simulink model "Prescan_Carsim_0118_repair_cs"  (R2019b)
settings: Solver=ode5  StartTime=0.0  StopTime=inf  FixedStep=1/1000  RelTol=1e-3
PreLoadFcn:
  | mbxruntime.callbacks.PreLoadFcn(bdroot);
PostLoadFcn:
  | mbxruntime.callbacks.PostLoadFcn(bdroot);
InitFcn:
  | mbxruntime.callbacks.InitFcn(bdroot);
  | Initialization_Func;
  | %T01_Init_2106;
StartFcn:
  | mbxruntime.callbacks.StartFcn(bdroot);
  | current_sys=gcs;
  | speedblock=Simulink.findBlocks(current_sys,'Name','speed_kmh_Gain');
  | h1=add_exec_event_listener(speedblock,'PostOutputs',@SpeedVisulization);
  | outblock=Simulink.findBlocks(current_sys,'Name','trajectorycurveoutput_Gain');
  | CurveTrajectoryListenerHandle=add_exec_event_listener(outblock,'PostOutputs',@TrajectoryCurve_CallBack);
  | lanedatablock=Simulink.findBlocks(current_sys,'Name','LaneData_Gain');
  | CurveLaneListenerHandle=add_exec_event_listener(lanedatablock,'PostOutputs',@CurveLane_CallBack);
StopFcn:
  | mbxruntime.callbacks.StopFcn(bdroot);
model workspace: external: MAT-File .\Prescan_Carsim_1230_cs_hws.mat (data not in the file)
undefined symbols (not defined in the file or in its folder): AAx, AAy, AAz, AVx, AVy, AVz, Ax, Ay, Az, canChannel, DiscIntNeverNeededParam, g, InitialDPMPDF_Comfort, InitialDPMPDF_Efficiency, InitialDPMPDF_Safety, InitialPDF_DEM, InitialPlanningParameter, Kf, Kr, Lr, M, mbxruntime, nG, NormalisedTrajectoryIndicator_Pool, Parameter_Indicator_LookUpTable, Prescan_Carsim_1230_cs_0658e9ca1334a8be, Prescan_Carsim_1230_cs_08c5eb9a1bd7376a, Prescan_Carsim_1230_cs_6cfd759b89b9fc85, Prescan_Carsim_1230_cs_9435cc1cceb5050d, Prescan_Carsim_1230_cs_ac716d34d49f74ab, Prescan_Carsim_1230_cs_be02757d7f212dd5, Rational_Coefficient_Learning, SteeringWheel, TrajectoryIndicatorRange, V, VehicleBaseLength, Vx, Vy, Vz, WheelL0, WheelL1, WheelR0, WheelR1
libraries: canmsglib x11, dsparch4 x6, canlib x3, PreScanSimulinkLibrary x3, Solver_SF x1, autolibshared x1
(part 2 of 8)

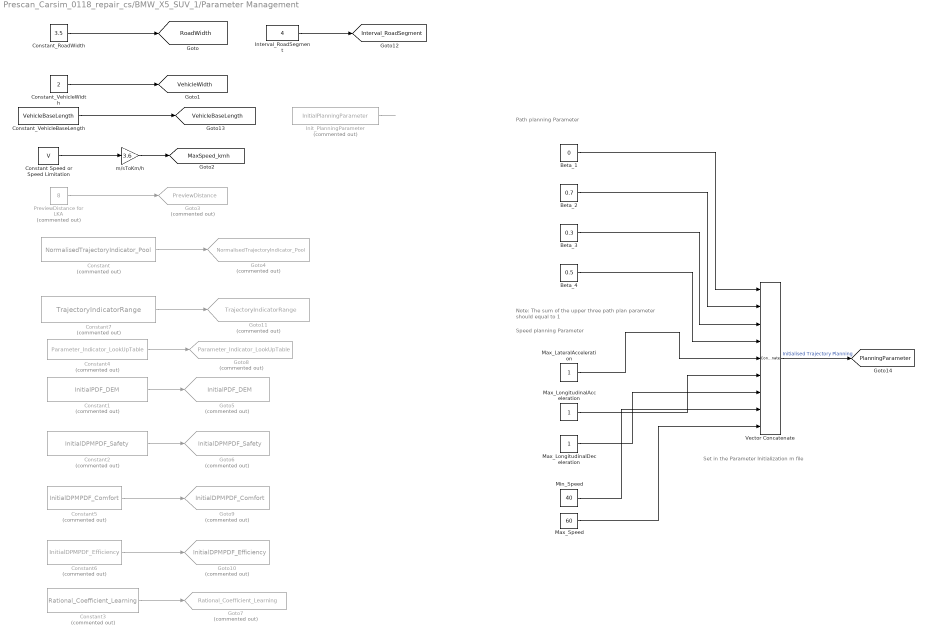
== system Prescan_Carsim_0118_repair_cs/BMW_X5_SUV_1/Parameter Management ==
  note: Set in the Parameter Initialization m file
  note: Note: The sum of the upper three path plan parameter should equal to 1
  note: Speed planning Parameter
  note: Path planning Parameter
  Beta_1 : Constant  Value=0
      settings: AttributesFormatString=|
      | weight of short path
      | within 0-1
  Beta_2 : Constant  Value=0.7
      settings: AttributesFormatString=|
      | weight of minimum curvature path
      | within 0-1
  Beta_3 : Constant  Value=0.3
      settings: AttributesFormatString=|
      | weight of fixed lateral offset
      | within 0-1
  Beta_4 : Constant  Value=0.5
      settings: AttributesFormatString=Fixed lateral offset distance
  Constant : Constant  Commented=on  Value=NormalisedTrajectoryIndicator_Pool
  Constant Speed or Speed Limitation : Constant  Value=V
  Constant1 : Constant  Commented=on  Value=InitialPDF_DEM
      settings: AttributesFormatString=|
      | The Initial probability density Distribution
      | of the S-C-E weight of the DEM
  Constant2 : Constant  Commented=on  Value=InitialDPMPDF_Safety
      settings: AttributesFormatString=|
      | The Initial probability density Distribution
      | of the DPM for S-C-E
  Constant3 : Constant  Commented=on  Value=Rational_Coefficient_Learning
  Constant4 : Constant  Commented=on  Value=Parameter_Indicator_LookUpTable
  Constant5 : Constant  Commented=on  Value=InitialDPMPDF_Comfort
      settings: AttributesFormatString=|
      | The Initial probability density Distribution
      | of the DPM for S-C-E
  Constant6 : Constant  Commented=on  Value=InitialDPMPDF_Efficiency
      settings: AttributesFormatString=|
      | The Initial probability density Distribution
      | of the DPM for S-C-E
  Constant7 : Constant  Commented=on  Value=TrajectoryIndicatorRange
  Constant_RoadWidth : Constant  Value=3.5
  Constant_VehicleBaseLength : Constant  Value=VehicleBaseLength
  Constant_VehicleWidth : Constant  Value=2
  Goto10 : Goto  Commented=on  GotoTag=InitialDPMPDF_Efficiency  TagVisibility=global
  Goto11 : Goto  Commented=on  GotoTag=TrajectoryIndicatorRange  TagVisibility=global
  Goto3 : Goto  Commented=on  GotoTag=PreviewDistance  TagVisibility=global
  Goto4 : Goto  Commented=on  GotoTag=NormalisedTrajectoryIndicator_Pool  TagVisibility=global
  Goto5 : Goto  Commented=on  GotoTag=InitialPDF_DEM  TagVisibility=global
  Goto6 : Goto  Commented=on  GotoTag=InitialDPMPDF_Safety  TagVisibility=global
  Goto7 : Goto  Commented=on  GotoTag=Rational_Coefficient_Learning  TagVisibility=global
  Goto8 : Goto  Commented=on  GotoTag=Parameter_Indicator_LookUpTable  TagVisibility=global
  Goto9 : Goto  Commented=on  GotoTag=InitialDPMPDF_Comfort  TagVisibility=global
  Init_PlanningParameter : Constant  Commented=on  Value=InitialPlanningParameter
  Interval_RoadSegment : Constant  Value=4
  Max_LateralAcceleration : Constant
      settings: AttributesFormatString=|
      | Maximum Lateral Acceleration (m/s2)
      | (within 0.5-2.5)
  Max_LongitudinalAcceleration : Constant
      settings: AttributesFormatString=|
      | Maximum Longitudinal Acceleration(m/s2)
      | ((within 0-3))
  Max_LongitudinalDeceleration : Constant
      settings: AttributesFormatString=|
      | Maximum Longitudinal Deceleration(m/s2)
      | (within 0-3)
  Max_Speed : Constant  Value=60
      settings: AttributesFormatString=Alowable Maximum Speed (Km/h)
  Min_Speed : Constant  Value=40
      settings: AttributesFormatString=Alowable Minimum Speed (Km/h)
  PreviewDistance for LKA : Constant  Commented=on  Value=8
  Vector Concatenate : Concatenate  NumInputs=9  Mode=Multidimensional array
  m/sToKm/h : Gain  Gain=3.6
  tag scope: Interval_RoadSegment=global, MaxSpeed_kmh=global, PlanningParameter=global, RoadWidth=global, VehicleBaseLength=global, VehicleWidth=global
  wires:
  m/sToKm/h/1 -> [MaxSpeed_kmh]
  PreviewDistance for LKA/1 -> Goto3/1
  Constant Speed or Speed Limitation/1 -> m/sToKm/h/1
  Constant_VehicleWidth/1 -> [VehicleWidth]
  Constant_RoadWidth/1 -> [RoadWidth]
  Constant/1 -> Goto4/1
  Constant1/1 -> Goto5/1
  Constant2/1 -> Goto6/1
  Constant3/1 -> Goto7/1
  Constant4/1 -> Goto8/1
  Constant5/1 -> Goto9/1
  Constant6/1 -> Goto10/1
  Constant7/1 -> Goto11/1
  Max_Speed/1 -> Vector Concatenate/9
  Max_LateralAcceleration/1 -> Vector Concatenate/5
  Beta_2/1 -> Vector Concatenate/2
  Max_LongitudinalDeceleration/1 -> Vector Concatenate/7
  Max_LongitudinalAcceleration/1 -> Vector Concatenate/6
  Beta_4/1 -> Vector Concatenate/4
  Min_Speed/1 -> Vector Concatenate/8
  Beta_1/1 -> Vector Concatenate/1
  Beta_3/1 -> Vector Concatenate/3
  Vector Concatenate/1 -> [PlanningParameter]  "Initialised Trajectory Planning"
  Interval_RoadSegment/1 -> [Interval_RoadSegment]
  Constant_VehicleBaseLength/1 -> [VehicleBaseLength]
  Init_PlanningParameter/1 -> ?

== system Prescan_Carsim_0118_repair_cs/BMW_X5_SUV_1/SELF_Demux ==
  SELF : Inport  OutDataTypeStr=Bus: PRESCAN_SELFSENSORDATA
  Bus Selector : BusSelector  OutputSignals=PositionX,PositionY,PositionZ,OrientationRoll,OrientationPitch,OrientationYaw,Velocity,Yaw_rate,Lat,Long,Alt,TimeStamp
  Demux2 : Demux  Outputs=3
  Gain : Gain  Gain=180/pi
  Gain1 : Gain  Gain=180/pi
  Vector Concatenate1 : Concatenate  NumInputs=3
  compas converter : Subsystem
  x [m] : Outport
  y [m] : Outport  Port=2
  z [m] : Outport  Port=3
  rotx [deg] : Outport  Port=4
  roty [deg] : Outport  Port=5
  rotz [deg] : Outport  Port=6
  GPS lat [deg] : Outport  Port=7
  GPS long [deg] : Outport  Port=8
  GPS alt [m] : Outport  Port=9
  velocity [m/s] : Outport  Port=10
  heading [deg] : Outport  Port=11
  yaw rate [deg/s] : Outport  Port=12
  TimeStamp [s] : Outport  Port=13
  wires:
  Bus Selector/12 -> TimeStamp [s]/1  "<TimeStamp>"
  Bus Selector/11 -> GPS alt [m]/1  "<Alt>"
  Bus Selector/10 -> GPS long [deg]/1  "<Long>"
  Bus Selector/9 -> GPS lat [deg]/1  "<Lat>"
  Bus Selector/8 -> Gain1/1  "<Yaw_rate>"
  Bus Selector/7 -> velocity [m/s]/1  "<Velocity>"
  Bus Selector/6 -> compas converter/1(rotz [rad]), Vector Concatenate1/3  "<OrientationYaw>"
  Bus Selector/5 -> Vector Concatenate1/2  "<OrientationPitch>"
  Bus Selector/4 -> Vector Concatenate1/1  "<OrientationRoll>"
  Vector Concatenate1/1 -> Gain/1
  Bus Selector/3 -> z [m]/1  "<PositionZ>"
  Bus Selector/2 -> y [m]/1  "<PositionY>"
  Bus Selector/1 -> x [m]/1  "<PositionX>"
  SELF/1 -> Bus Selector/1
  Gain/1 -> Demux2/1
  Demux2/1 -> rotx [deg]/1
  Demux2/2 -> roty [deg]/1
  Demux2/3 -> rotz [deg]/1
  compas converter/1(heading [deg]) -> heading [deg]/1
  Gain1/1 -> yaw rate [deg/s]/1

== system Prescan_Carsim_0118_repair_cs/BMW_X5_SUV_1/STATE_BMW_X5_SUV_1 ==
  State : Inport  SampleTime=TimeStep
  Bus Creator : BusCreator  Inputs=15  OutDataTypeStr=Bus: PRESCAN_STATEACTUATORDATA  NonVirtualBus=on
  Constant : Constant  Value=0
  Demux : Demux  Outputs=15
  Mux : Mux  Inputs=3
  Mux1 : Mux  Inputs=3
  Mux2 : Mux  Inputs=3
  iniBODYAngles wrtVEH [rad] : Constant  Value=Roll0  SampleTime=TimeStep
  iniBODYAngles wrtVEH [rad]1 : Constant  Value=Pitch0  SampleTime=TimeStep
  iniVEHAngles wrtGLOB [rad] : Constant  Value=Yaw0  SampleTime=TimeStep
  iniVEHposition wrtGLOB [m] : Constant  Value=x0  SampleTime=TimeStep
  iniVEHposition wrtGLOB [m]1 : Constant  Value=y0  SampleTime=TimeStep
  iniVEHposition wrtGLOB [m]2 : Constant  Value=z0  SampleTime=TimeStep
  state2FullState : PreScanSimulinkLibrary/state2FullState  SystemSampleTime=-1  Latency=0  AutoFrameSizeCalculation=off
  StateBus : Outport  OutDataTypeStr=Bus: PRESCAN_STATEACTUATORDATA
  wires:
  Bus Creator/1 -> StateBus/1
  State/1 -> state2FullState/1
  state2FullState/1 -> Demux/1
  Demux/1 -> Bus Creator/1  "PositionX"
  Demux/2 -> Bus Creator/2  "PositionY"
  Demux/3 -> Bus Creator/3  "PositionZ"
  Demux/4 -> Bus Creator/4  "VelocityX"
  Demux/5 -> Bus Creator/5  "VelocityY"
  Demux/6 -> Bus Creator/6  "VelocityZ"
  Demux/7 -> Bus Creator/7  "AccelerationX"
  Demux/8 -> Bus Creator/8  "AccelerationY"
  Demux/9 -> Bus Creator/9  "AccelerationZ"
  Demux/10 -> Bus Creator/10  "OrientationRoll"
  Demux/11 -> Bus Creator/11  "OrientationPitch"
  Demux/12 -> Bus Creator/12  "OrientationYaw"
  Demux/13 -> Bus Creator/13  "AngularVelocityRoll"
  Demux/14 -> Bus Creator/14  "AngularVelocityPitch"
  Demux/15 -> Bus Creator/15  "AngularVelocityYaw"
  iniVEHposition wrtGLOB [m]1/1 -> Mux/2
  iniVEHposition wrtGLOB [m]/1 -> Mux/1
  iniVEHposition wrtGLOB [m]2/1 -> Mux/3
  Mux/1 -> state2FullState/2
  iniBODYAngles wrtVEH [rad]/1 -> Mux1/1
  iniBODYAngles wrtVEH [rad]1/1 -> Mux1/2
  Constant/1 -> Mux1/3, Mux2/2, Mux2/1
  Mux1/1 -> state2FullState/3
  iniVEHAngles wrtGLOB [rad]/1 -> Mux2/3
  Mux2/1 -> state2FullState/4

== system Prescan_Carsim_0118_repair_cs/BMW_X5_SUV_1/SteeringWheel_pivot_Mux ==
  X [m] : Inport
  Y [m] : Inport  Port=2
  Z [m] : Inport  Port=3
  Roll [rad] : Inport  Port=4
  Pitch [rad] : Inport  Port=5
  Yaw [rad] : Inport  Port=6
  Bus Creator : BusCreator  Inputs=3  OutDataTypeStr=Bus: PRESCAN_XYZ_DATA
  Bus Creator1 : BusCreator  Inputs=3  OutDataTypeStr=Bus: PRESCAN_RPY_DATA
  Bus Creator2 : BusCreator  Inputs=2  OutDataTypeStr=Bus: PRESCAN_POSE_DATA
  Joint : Outport
  wires:
  Yaw [rad]/1 -> Bus Creator1/3  "Yaw"
  Bus Creator1/1 -> Bus Creator2/2  "ORIENTATION"
  Bus Creator/1 -> Bus Creator2/1  "POSITION"
  X [m]/1 -> Bus Creator/1  "X"
  Y [m]/1 -> Bus Creator/2  "Y"
  Z [m]/1 -> Bus Creator/3  "Z"
  Bus Creator2/1 -> Joint/1
  Roll [rad]/1 -> Bus Creator1/1  "Roll"
  Pitch [rad]/1 -> Bus Creator1/2  "Pitch"

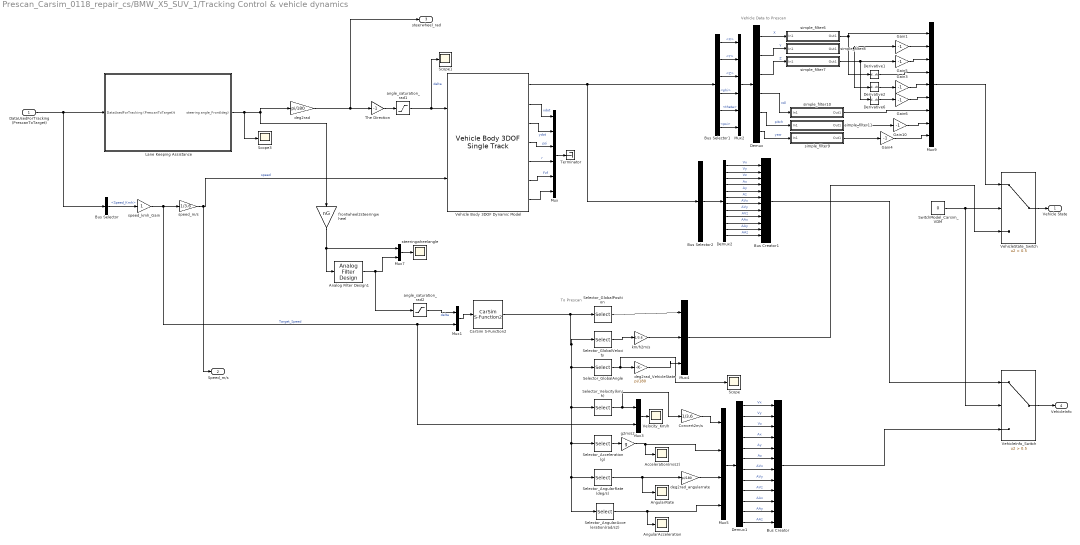
== system Prescan_Carsim_0118_repair_cs/BMW_X5_SUV_1/Tracking Control & vehicle dynamics ==
  note: To Prescan
  note: Vehicle Data to Prescan
  DataUsedForTracking (PrescanToTarget) : Inport
  Acceleration(m/s2) : Scope
  Analog Filter Design1 : dsparch4/Analog Filter Design  method=Butterworth  filttype=Lowpass  N=1  Wlo=5  Whi=80  Rp=2  Rs=40
  AngularAcceleration : Scope
  AngularRate : Scope
  Bus Creator : BusCreator  Inputs=Vx,Vy,Vz,Ax,Ay,Az,AVx,AVy,AVz,AAx,AAy,AAz
  Bus Creator1 : BusCreator  Inputs=Vx,Vy,Vz,Ax,Ay,Az,AVx,AVy,AVz,AAx,AAy,AAz
  Bus Selector : BusSelector  OutputSignals=Speed_Kmh
  Bus Selector1 : BusSelector  OutputSignals=InertFrm.Cg.Disp.X,InertFrm.Cg.Disp.Y,InertFrm.Cg.Disp.Z,InertFrm.Cg.Ang.phi,InertFrm.Cg.Ang.theta,InertFrm.Cg.Ang.psi
  Bus Selector2 : BusSelector  OutputSignals=BdyFrm.Cg.Vel.xdot,BdyFrm.Cg.Vel.ydot,BdyFrm.Cg.Vel.zdot,BdyFrm.Cg.Acc.xddot,BdyFrm.Cg.Acc.yddot,BdyFrm.Cg.Acc.zddot,BdyFrm.Cg.AngVel.p,BdyFrm.Cg.AngVel.q,BdyFrm.Cg.AngVel.r,BdyFrm.Cg.AngAcc.pdot,BdyFrm.Cg.AngAcc.qdot,BdyFrm.Cg.AngAcc.rdot  OutputAsBus=on
  CarSim S-Function2 : Solver_SF/CarSim S-Function2  Priority=1  VehicleCode=i_i  SIMFILE=simfile.sim
      settings: SourceProductName=CarSim S-Function
      settings: AttributesFormatString=|
      | Vehicle Code: %<VehicleCode>
      | Input:Steering Wheel Angel(deg)
      | 2,Speed(km/h)
      | Output:
      | 1,X,Y,Z(m)
      | 2,Roll,Pitch,Yaw(deg)
      | 3,Longitudinal and Lateral Acceleration(g)
      | 4,Roll,Pitch and Yaw rate (deg/s)
      | 5,Roll and Yaw acceleration (rad/s2)
      | 6,SteeringWheelAngel and 4 Wheels Angle(deg)
  Convert2m/s : Gain  Gain=1/3.6
  Demux : Demux  Outputs=6
  Demux1 : Demux  Outputs=12
  Demux2 : Demux  Outputs=12  BusSelectionMode=on
  Derivative1 : Derivative
  Derivative2 : Derivative
  Derivative6 : Derivative
  Gain{1,3..6,10} (6 alike) : Gain  Gain=-1
  Lane Keeping Assistance : Subsystem
  Mux : Mux  Inputs=6
  Mux1 : Mux  Inputs=2
  Mux2 : Mux  Inputs=6
  Mux3 : Mux  Inputs=2
  Mux4 : Mux  Inputs=3
  Mux5 : Mux
  Mux7 : Mux  Inputs=2
  Mux9 : Mux  Inputs=9
  Scope : Scope
  Scope1 : Scope
  Scope3 : Scope
  Selector_Acceleration(g) : Selector  InputPortWidth=21  IndexOptions=Index vector (dialog)  Indices=[13:15]  OutputSizes=1
  Selector_AngularAcceleration(rad/s2) : Selector  InputPortWidth=21  IndexOptions=Index vector (dialog)  Indices=[19:21]  OutputSizes=1
  Selector_AngularRate(deg/s) : Selector  InputPortWidth=21  IndexOptions=Index vector (dialog)  Indices=[16:18]  OutputSizes=1
  Selector_GlobalAngle : Selector  InputPortWidth=21  IndexOptions=Index vector (dialog)  Indices=[7:9]  OutputSizes=1
  Selector_GlobalPosition : Selector  InputPortWidth=21  IndexOptions=Index vector (dialog)  Indices=[1:3]  OutputSizes=1
  Selector_GlobalVelocity : Selector  InputPortWidth=21  IndexOptions=Index vector (dialog)  Indices=[4:6]  OutputSizes=1
  Selector_Velocity(km/h) : Selector  InputPortWidth=21  IndexOptions=Index vector (dialog)  Indices=[10:12]  OutputSizes=1
  SwitchModel_Carsim_VDM : Constant  Value=0
      settings: AttributesFormatString=|
      | 0:Carsim
      | 1:Simulink VDM
  Terminator : Terminator
  "The Direction " : Gain  Gain=-1
  Vehicle Body 3DOF Dynamic Model : autolibshared/Vehicle Body 3DOF Single Track  trackMode=Single (bicycle)  inputMode=External longitudinal velocity  frontSteerMode=on  rearSteerMode=off  windMode=off  muMode=off  extFMode=off  extMMode=off  extXo=off  extpsio=off  extxdoto=off  extro=off  extYo=off  extTamb=off  extydoto=off  aMode=2  NF=2  NR=2  m=M  a=Lf  b=Lr  h=0.35  X_o=0  xdot_o=0  CalphaMode=off  sigmaMode=off  d=0  w=[1.4,1.4]  Cy_f=Kf*2  Cy_r=Kr*2  sigma_f=.1  sigma_r=.1  alpha_f_brk=[-.1 .1]  Cy_f_data=[-9e3 9e3]  alpha_r_brk=[-.1 .1]  Cy_r_data=[-9e3 9e3]  Y_o=0  ydot_o=0  Izz=I  psi_o=0  r_o=0  Af=0  Cd=.3  Cl=.1  Cpm=.1  beta_w=[0:0.01:0.3]  Cs=[0:0.03:0.9]  Cym=[0:0.01:0.3]  Pabs=101325  Tair=273  g=g  mu=1  xdot_tol=.01  Fznom=5000  Fxtire_sat=7e4  Fytire_sat=7e4  longOff=0  latOff=0  vertOff=0  wrapAng=off
      settings: SourceProductBaseCode=PW,MT,VE,VP
  VehicleInfo_Switch : Switch  Criteria=u2 > Threshold  Threshold=0.5
  VehicleState_Switch : Switch  Criteria=u2 > Threshold  Threshold=0.5
  Velocity_Km/h : Scope
  angle_saturation_rad1 : Saturate  UpperLimit=1.5  LowerLimit=-1.5
  angle_saturation_rad2 : Saturate  UpperLimit=86  LowerLimit=-86
  deg2rad : Gain  Gain=pi/180
  deg2rad_VehicleState : Gain  Gain=pi/180
  deg2rad_angularrate : Gain  Gain=pi/180
  frontwheel2steeringwheel : Gain  Gain=nG
      settings: AttributesFormatString=Calculatedd by the carsim table
  g2m/s2 : Gain  Gain=g
  km/h2m/s : Gain  Gain=1/3.6
  simple_filter10 : Subsystem
  simple_filter11 : Subsystem
  simple_filter6 : Subsystem
  simple_filter7 : Subsystem
  simple_filter8 : Subsystem
  simple_filter9 : Subsystem
  speed_kmh_Gain : Gain
  speed_m/s : Gain  Gain=1/3.6
  steeringwheelangle : Scope
  Vehicle State : Outport
  Speed_m/s : Outport  Port=2
  "steerwheel_rad " : Outport  Port=3
  VehicleInfo : Outport  Port=4
  wires:
  "The Direction "/1 -> angle_saturation_rad1/1
  Mux/1 -> Terminator/1
  Vehicle Body 3DOF Dynamic Model/7 -> Mux/6
  Vehicle Body 3DOF Dynamic Model/6 -> Mux/5  "Fzf"
  Vehicle Body 3DOF Dynamic Model/5 -> Mux/4  "r"
  Vehicle Body 3DOF Dynamic Model/4 -> Mux/3  "psi"
  Vehicle Body 3DOF Dynamic Model/3 -> Mux/2  "ydot"
  Vehicle Body 3DOF Dynamic Model/2 -> Mux/1  "xdot"
  angle_saturation_rad1/1 -> Scope1/1, Vehicle Body 3DOF Dynamic Model/1  "delta"
  deg2rad/1 -> "steerwheel_rad "/1, "The Direction "/1
  DataUsedForTracking (PrescanToTarget)/1 -> Bus Selector/1, Lane Keeping Assistance/1(DataUsedForTracking (PrescanToTarget)t)
  Bus Selector1/3 -> Mux2/3  "<Z>"
  simple_filter9/1(Out1) -> Gain4/1
  Bus Selector1/5 -> Mux2/5  "<theta>"
  Gain4/1 -> Mux9/9
  Demux/5 -> simple_filter11/1(In1)  "pitch"
  simple_filter8/1(Out1) -> Derivative2/1, Gain1/1
  Demux/6 -> simple_filter9/1(In1)  "yaw"
  Gain6/1 -> Mux9/6
  simple_filter6/1(Out1) -> Derivative1/1, Mux9/1
  Gain1/1 -> Mux9/2
  Gain3/1 -> Mux9/5
  Gain10/1 -> Mux9/8
  Bus Selector1/2 -> Mux2/2  "<Y>"
  Derivative1/1 -> Mux9/4
  Demux/4 -> simple_filter10/1(In1)  "roll"
  Derivative6/1 -> Gain6/1
  simple_filter7/1(Out1) -> Derivative6/1, Gain5/1
  Demux/3 -> simple_filter7/1(In1)  "Z"
  Derivative2/1 -> Gain3/1
  simple_filter10/1(Out1) -> Mux9/7
  Demux/1 -> simple_filter6/1(In1)  "X"
  Bus Selector1/4 -> Mux2/4  "<phi>"
  Bus Selector1/6 -> Mux2/6  "<psi>"
  Demux/2 -> simple_filter8/1(In1)  "Y"
  Mux2/1 -> Demux/1
  simple_filter11/1(Out1) -> Gain10/1
  Bus Selector1/1 -> Mux2/1  "<X>"
  Gain5/1 -> Mux9/3
  Mux9/1 -> VehicleState_Switch/1
  speed_m/s/1 -> Speed_m/s/1, Vehicle Body 3DOF Dynamic Model/2  "speed"
  Bus Selector/1 -> speed_kmh_Gain/1  "<Speed_Kmh>"
  Lane Keeping Assistance/1(steering angle_Front(deg)) -> Scope3/1, frontwheel2steeringwheel/1, deg2rad/1
  Selector_GlobalAngle/1 -> Scope/1, deg2rad_VehicleState/1
  km/h2m/s/1 -> Mux4/2
  Selector_GlobalVelocity/1 -> km/h2m/s/1
  Selector_GlobalPosition/1 -> Mux4/1
  Mux1/1 -> CarSim S-Function2/1
  deg2rad_VehicleState/1 -> Mux4/3
  Mux4/1 -> VehicleState_Switch/3
  VehicleState_Switch/1 -> Vehicle State/1
  angle_saturation_rad2/1 -> Mux1/1  "delta"
  Mux7/1 -> steeringwheelangle/1
  Analog Filter Design1/1 -> angle_saturation_rad2/1, Mux7/2
  frontwheel2steeringwheel/1 -> Mux7/1, Analog Filter Design1/1
  SwitchModel_Carsim_VDM/1 -> VehicleInfo_Switch/2, VehicleState_Switch/2
  VehicleInfo_Switch/1 -> VehicleInfo/1
  Selector_AngularRate(deg/s)/1 -> AngularRate/1, deg2rad_angularrate/1
  Selector_AngularAcceleration(rad/s2)/1 -> Mux5/4, AngularAcceleration/1
  Selector_Acceleration(g)/1 -> g2m/s2/1
  g2m/s2/1 -> Mux5/2, Acceleration(m/s2)/1
  Mux3/1 -> Velocity_Km/h/1
  CarSim S-Function2/1 -> Selector_AngularAcceleration(rad/s2)/1, Selector_AngularRate(deg/s)/1, Selector_Acceleration(g)/1, Selector_Velocity(km/h)/1, Selector_GlobalAngle/1, Selector_GlobalVelocity/1, Selector_GlobalPosition/1
  Selector_Velocity(km/h)/1 -> Convert2m/s/1, Mux3/1
  Convert2m/s/1 -> Mux5/1
  Bus Creator/1 -> VehicleInfo_Switch/3
  Mux5/1 -> Demux1/1
  Demux1/9 -> Bus Creator/9  "AVz"
  Demux1/8 -> Bus Creator/8  "AVy"
  Demux1/7 -> Bus Creator/7  "AVx"
  Demux1/5 -> Bus Creator/5  "Ay"
  Demux1/4 -> Bus Creator/4  "Ax"
  Demux1/3 -> Bus Creator/3  "Vz"
  Demux1/2 -> Bus Creator/2  "Vy"
  Demux1/1 -> Bus Creator/1  "Vx"
  Demux1/6 -> Bus Creator/6  "Az"
  Demux1/10 -> Bus Creator/10  "AAx"
  Demux1/11 -> Bus Creator/11  "AAy"
  Demux1/12 -> Bus Creator/12  "AAz"
  Bus Selector2/1 -> Demux2/1
  Demux2/1 -> Bus Creator1/1  "Vx"
  Demux2/2 -> Bus Creator1/2  "Vy"
  Demux2/3 -> Bus Creator1/3  "Vz"
  Demux2/4 -> Bus Creator1/4  "Ax"
  Demux2/5 -> Bus Creator1/5  "Ay"
  Demux2/6 -> Bus Creator1/6  "Az"
  Demux2/7 -> Bus Creator1/7  "AVx"
  Demux2/8 -> Bus Creator1/8  "AVy"
  Demux2/9 -> Bus Creator1/9  "AVz"
  Demux2/10 -> Bus Creator1/10  "AAx"
  Demux2/11 -> Bus Creator1/11  "AAy"
  Demux2/12 -> Bus Creator1/12  "AAz"
  Bus Creator1/1 -> VehicleInfo_Switch/1
  speed_kmh_Gain/1 -> Mux3/2, Mux1/2, speed_m/s/1  "Target_Speed"
  Vehicle Body 3DOF Dynamic Model/1 -> Bus Selector2/1, Bus Selector1/1
  deg2rad_angularrate/1 -> Mux5/3

== system Prescan_Carsim_0118_repair_cs/BMW_X5_SUV_1/Trajectory Indicator Calculation ==
  note: For TLC Calculation
  note: Vehicle Information During Curve
  Vehicle_Info : Inport
      settings: AttributesFormatString=Specified Sample Time 1/20
  Bus Selector3 : BusSelector  OutputSignals=Vx,Vy,Vz,Ax,Ay,Az,AVx,AVy,AVz,AAx,AAy,AAz
  Clock : Clock
  From3 : From  Commented=on  GotoTag=TLC_Left  TagVisibility=global
  From4 : From  Commented=on  GotoTag=TLC_Right  TagVisibility=global
  Rate Transition1 : RateTransition  OutPortSampleTime=1/20
      settings: AttributesFormatString=|
      | Set the Sample Frequency for the vehicle
      | Information durving curve
  Rate Transition2 : RateTransition  OutPortSampleTime=1/20
      settings: AttributesFormatString=|
      | Set the Sample Frequency for the vehicle
      | Information durving curve
  Rate Transition3 : RateTransition  OutPortSampleTime=1/20
      settings: AttributesFormatString=|
      | Set the Sample Frequency for the vehicle
      | Information durving curve
  To File : ToFile  Filename=TrajectoryCurve.mat  MatrixName=Trajectory  SaveFormat=Timeseries
      settings: Decimation=10000
  Vector Concatenate : Concatenate  NumInputs=15  Mode=Multidimensional array  ConcatenateDimension=2
  VehicleInfo_Curve : Subsystem  TreatAsAtomicUnit=on
      settings: AttributesFormatString=output the Vehicle Info when exit the curve
  VehicleState_Buffer : Subsystem  TreatAsAtomicUnit=on
  tag scope: Speed_Rel=global, YawRate=global
  wires:
  Rate Transition1/1 -> Bus Selector3/1
  [Curve_Flag] -> VehicleInfo_Curve/Trigger, VehicleState_Buffer/Enable
  VehicleState_Buffer/1(VehicleInfo_Curve) -> VehicleInfo_Curve/1(In1)
  Vector Concatenate/1 -> VehicleState_Buffer/1(In1)
  Vehicle_Info/1 -> Rate Transition1/1
  VehicleInfo_Curve/1(VehicleInfo_Curve) -> To File/1
  [LateralOffset] -> Rate Transition3/1
  Clock/1 -> Rate Transition2/1
  Rate Transition2/1 -> Vector Concatenate/1
  Rate Transition3/1 -> Vector Concatenate/14
  Bus Selector3/1 -> [Speed_Rel], Vector Concatenate/2  "<Vx>"
  Bus Selector3/2 -> Vector Concatenate/3  "<Vy>"
  Bus Selector3/3 -> Vector Concatenate/4  "<Vz>"
  Bus Selector3/4 -> Vector Concatenate/5  "<Ax>"
  Bus Selector3/5 -> Vector Concatenate/6  "<Ay>"
  Bus Selector3/6 -> Vector Concatenate/7  "<Az>"
  Bus Selector3/7 -> Vector Concatenate/8  "<AVx>"
  Bus Selector3/8 -> Vector Concatenate/9  "<AVy>"
  Bus Selector3/9 -> Vector Concatenate/10  "<AVz>"
  Bus Selector3/10 -> [YawRate], Vector Concatenate/11  "<AAx>"
  Bus Selector3/11 -> Vector Concatenate/12  "<AAy>"
  Bus Selector3/12 -> Vector Concatenate/13  "<AAz>"
  [VehicleState_Global] -> Vector Concatenate/15

== system Prescan_Carsim_0118_repair_cs/BMW_X5_SUV_1/VehicleToPrescan ==
  note: Vehicle Data to Prescan
  Vehicle Info : Inport
  Bus Selector1 : BusSelector  OutputSignals=InertFrm.Cg.Disp.X,InertFrm.Cg.Disp.Y,InertFrm.Cg.Disp.Z,InertFrm.Cg.Ang.phi,InertFrm.Cg.Ang.theta,InertFrm.Cg.Ang.psi
  Derivative1 : Derivative
  Derivative2 : Derivative
  Derivative6 : Derivative
  Gain{1,3..6,10} (6 alike) : Gain  Gain=-1
  Mux9 : Mux  Inputs=9
  simple_filter10 : Subsystem
  simple_filter11 : Subsystem
  simple_filter6 : Subsystem
  simple_filter7 : Subsystem
  simple_filter8 : Subsystem
  simple_filter9 : Subsystem
  VehicleStateToPrescan : Outport
  wires:
  Mux9/1 -> VehicleStateToPrescan/1
  Bus Selector1/5 -> simple_filter11/1(In1)  "<theta>"
  Gain10/1 -> Mux9/8
  simple_filter9/1(Out1) -> Gain4/1
  Derivative1/1 -> Mux9/4
  Bus Selector1/1 -> simple_filter6/1(In1)  "<X>"
  simple_filter11/1(Out1) -> Gain10/1
  Vehicle Info/1 -> Bus Selector1/1
  Bus Selector1/6 -> simple_filter9/1(In1)  "<psi>"
  simple_filter8/1(Out1) -> Gain1/1, Derivative2/1
  simple_filter10/1(Out1) -> Mux9/7
  Gain3/1 -> Mux9/5
  Gain4/1 -> Mux9/9
  Gain5/1 -> Mux9/3
  Bus Selector1/4 -> simple_filter10/1(In1)  "<phi>"
  Bus Selector1/3 -> simple_filter7/1(In1)  "<Z>"
  Bus Selector1/2 -> simple_filter8/1(In1)  "<Y>"
  Gain1/1 -> Mux9/2
  simple_filter7/1(Out1) -> Derivative6/1, Gain5/1
  simple_filter6/1(Out1) -> Derivative1/1, Mux9/1
  Gain6/1 -> Mux9/6
  Derivative2/1 -> Gain3/1
  Derivative6/1 -> Gain6/1

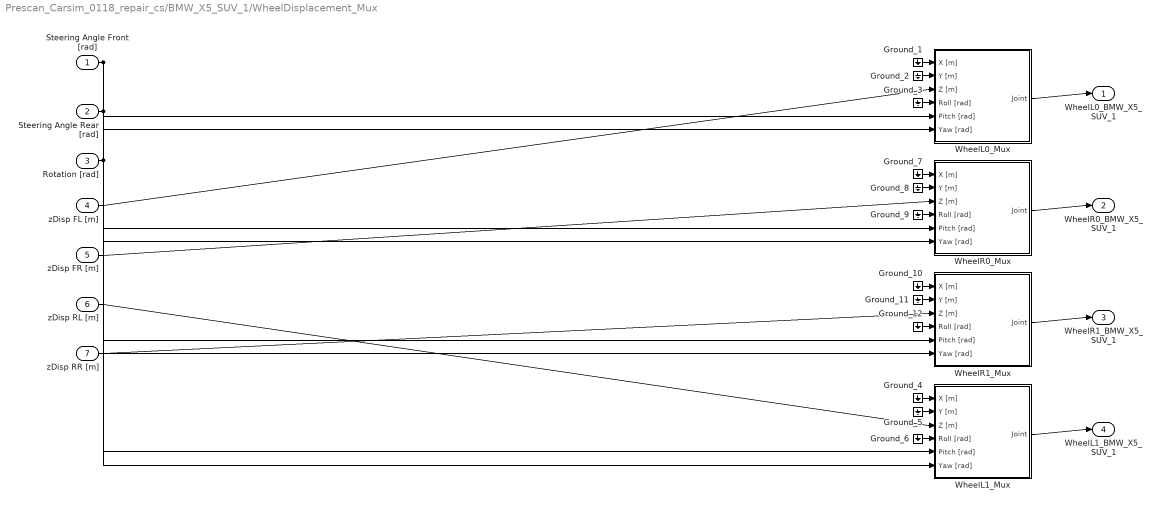
== system Prescan_Carsim_0118_repair_cs/BMW_X5_SUV_1/WheelDisplacement_Mux ==
  Steering Angle Front [rad] : Inport  Tag=inport/JointGroup  SampleTime=50/1000  BusOutputAsStruct=on
  Steering Angle Rear [rad] : Inport  Tag=inport/JointGroup  Port=2  SampleTime=50/1000  BusOutputAsStruct=on
  Rotation [rad] : Inport  Tag=inport/JointGroup  Port=3  SampleTime=50/1000  BusOutputAsStruct=on
  zDisp FL [m] : Inport  Tag=inport/JointGroup  Port=4  SampleTime=50/1000  BusOutputAsStruct=on
  zDisp FR [m] : Inport  Tag=inport/JointGroup  Port=5  SampleTime=50/1000  BusOutputAsStruct=on
  zDisp RL [m] : Inport  Tag=inport/JointGroup  Port=6  SampleTime=50/1000  BusOutputAsStruct=on
  zDisp RR [m] : Inport  Tag=inport/JointGroup  Port=7  SampleTime=50/1000  BusOutputAsStruct=on
  Ground_{1..12} (12 alike) : Ground
  WheelL0_Mux : Subsystem  Tag=mux/Joint  mask(PreScan Mux Block){DisplayName=WheelL0}
      mask prompts: DisplayName "Display Name"
      mask help:
      | This block simulates a generic joint used for generic models. This joint can be enabled/disabled from the GUI.
      |
      | For more information, please click Help.
      settings: DeleteFcn=PreScanBlockDeleteFcn;
      mask Help: eval('openHelp(254)')
  WheelL1_Mux : Subsystem  Tag=mux/Joint  mask(PreScan Mux Block){DisplayName=WheelL1}
      mask prompts: DisplayName "Display Name"
      mask help:
      | This block simulates a generic joint used for generic models. This joint can be enabled/disabled from the GUI.
      |
      | For more information, please click Help.
      settings: DeleteFcn=PreScanBlockDeleteFcn;
      mask Help: eval('openHelp(254)')
  WheelR0_Mux : Subsystem  Tag=mux/Joint  mask(PreScan Mux Block){DisplayName=WheelR0}
      mask prompts: DisplayName "Display Name"
      mask help:
      | This block simulates a generic joint used for generic models. This joint can be enabled/disabled from the GUI.
      |
      | For more information, please click Help.
      settings: DeleteFcn=PreScanBlockDeleteFcn;
      mask Help: eval('openHelp(254)')
  WheelR1_Mux : Subsystem  Tag=mux/Joint  mask(PreScan Mux Block){DisplayName=WheelR1}
      mask prompts: DisplayName "Display Name"
      mask help:
      | This block simulates a generic joint used for generic models. This joint can be enabled/disabled from the GUI.
      |
      | For more information, please click Help.
      settings: DeleteFcn=PreScanBlockDeleteFcn;
      mask Help: eval('openHelp(254)')
  WheelL0_BMW_X5_SUV_1 : Outport  Tag=outport/JointActuator  OutDataTypeStr=Bus: PRESCAN_POSE_DATA  SampleTime=50/1000
  WheelR0_BMW_X5_SUV_1 : Outport  Tag=outport/JointActuator  Port=2  OutDataTypeStr=Bus: PRESCAN_POSE_DATA  SampleTime=50/1000
  WheelR1_BMW_X5_SUV_1 : Outport  Tag=outport/JointActuator  Port=3  OutDataTypeStr=Bus: PRESCAN_POSE_DATA  SampleTime=50/1000
  WheelL1_BMW_X5_SUV_1 : Outport  Tag=outport/JointActuator  Port=4  OutDataTypeStr=Bus: PRESCAN_POSE_DATA  SampleTime=50/1000
  wires:
  WheelL0_Mux/1(Joint) -> WheelL0_BMW_X5_SUV_1/1
  WheelR0_Mux/1(Joint) -> WheelR0_BMW_X5_SUV_1/1
  WheelR1_Mux/1(Joint) -> WheelR1_BMW_X5_SUV_1/1
  WheelL1_Mux/1(Joint) -> WheelL1_BMW_X5_SUV_1/1
  Steering Angle Front [rad]/1 -> WheelR0_Mux/6(Yaw [rad]), WheelL0_Mux/6(Yaw [rad])
  Steering Angle Rear [rad]/1 -> WheelR1_Mux/6(Yaw [rad]), WheelL1_Mux/6(Yaw [rad])
  Rotation [rad]/1 -> WheelR0_Mux/5(Pitch [rad]), WheelL0_Mux/5(Pitch [rad]), WheelR1_Mux/5(Pitch [rad]), WheelL1_Mux/5(Pitch [rad])
  zDisp FL [m]/1 -> WheelL0_Mux/3(Z [m])
  zDisp FR [m]/1 -> WheelR0_Mux/3(Z [m])
  zDisp RL [m]/1 -> WheelL1_Mux/3(Z [m])
  zDisp RR [m]/1 -> WheelR1_Mux/3(Z [m])
  Ground_1/1 -> WheelL0_Mux/1(X [m])
  Ground_2/1 -> WheelL0_Mux/2(Y [m])
  Ground_3/1 -> WheelL0_Mux/4(Roll [rad])
  Ground_4/1 -> WheelL1_Mux/1(X [m])
  Ground_5/1 -> WheelL1_Mux/2(Y [m])
  Ground_6/1 -> WheelL1_Mux/4(Roll [rad])
  Ground_7/1 -> WheelR0_Mux/1(X [m])
  Ground_8/1 -> WheelR0_Mux/2(Y [m])
  Ground_9/1 -> WheelR0_Mux/4(Roll [rad])
  Ground_10/1 -> WheelR1_Mux/1(X [m])
  Ground_11/1 -> WheelR1_Mux/2(Y [m])
  Ground_12/1 -> WheelR1_Mux/4(Roll [rad])

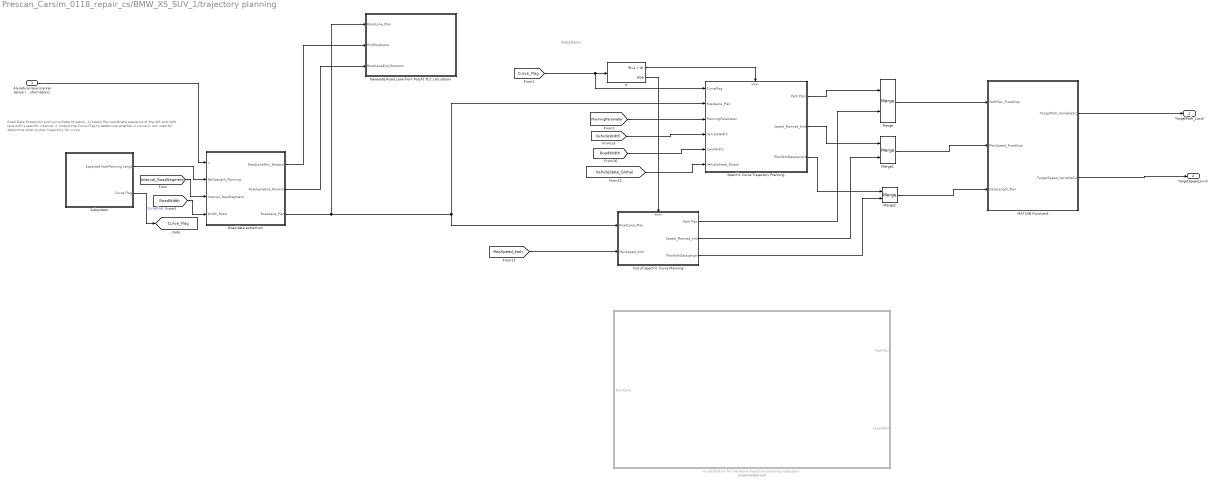
== system Prescan_Carsim_0118_repair_cs/BMW_X5_SUV_1/trajectory planning ==
  note: Subsystem1
  note: Road Data Extraction and Curve Determination,
      | 1,Output the coordinate sequence of the left and right lane with a specific interval;
      | 2, Output the Curve Flag to determine whether in curve or not, used for determine when to plan trajectory for curve
  Alynatical lane marker sensor information1 : Inport
  A substitution for the above trajectory planning subsystem : Subsystem  Commented=on
  "Generate Road Lane from Polyfit TLC calculation " : Subsystem
  If : If
  MATLAB Function1 : MATLAB Function  TreatAsAtomicUnit=on  SystemSampleTime=1/20
      settings: AttributesFormatString=|
      | Convert Variable Size into Fixed Size
      | Specified Sample Time:1/20
  Merge : Merge
  Merge1 : Merge
  Merge2 : Merge
  Out of Specific Curve Planning : Subsystem  TreatAsAtomicUnit=on
  Road data extraction : MATLAB Function  TreatAsAtomicUnit=on
  Specific Curve Trajectory Planning : Subsystem  TreatAsAtomicUnit=on
  Subsystem : Subsystem
      settings: AttributesFormatString=Determine the Planned Path length
  TargetPath_Local : Outport
      settings: AttributesFormatString=|
      | A fixed Length 1000
      | Valid Length PlanPathDataLength
  TargetSpeed_kmh : Outport  Port=2
      settings: AttributesFormatString=|
      | A fixed Length 1000
      | Valid Length PlanPathDataLength
  tag scope: Curve_Flag=global
  wires:
  [RoadWidth] -> Road data extraction/4(Width_Road)
  Subsystem/1(Expected PathPlanning Length) -> Road data extraction/2(PathLength_Planning)
  Subsystem/2(Curve Flag) -> [Curve_Flag]  "CurveFlag"
  Alynatical lane marker sensor information1/1 -> Road data extraction/1(u)
  [Interval_RoadSegment] -> Road data extraction/3(Interval_RoadSegment)
  Merge/1 -> MATLAB Function1/1(PathPlan_FixedSize)
  Out of Specific Curve Planning/1(Path Plan) -> Merge/2
  Specific Curve Trajectory Planning/1(Path Plan) -> Merge/1
  If/2 -> Out of Specific Curve Planning/Action
  If/1 -> Specific Curve Trajectory Planning/Action
  [Curve_Flag] -> Specific Curve Trajectory Planning/1(CurveFlag), If/1
  Specific Curve Trajectory Planning/2(Speed_Planned_kmh) -> Merge1/1
  Out of Specific Curve Planning/2(Speed_Planned_kmh) -> Merge1/2
  Merge1/1 -> MATLAB Function1/2(PlanSpeed_FixedSize)
  Specific Curve Trajectory Planning/3(PlanPathDataLength) -> Merge2/1
  Out of Specific Curve Planning/3(PlanPathDataLength) -> Merge2/2
  Merge2/1 -> MATLAB Function1/3(DataLength_Plan)
  [RoadWidth] -> Specific Curve Trajectory Planning/5(LaneWidth)
  [VehicleWidth] -> Specific Curve Trajectory Planning/4(VehicleWidth)
  [VehicleState_Global] -> Specific Curve Trajectory Planning/6(VehicleState_Global)
  [MaxSpeed_kmh] -> Out of Specific Curve Planning/2(MaxSpeed_Kmh)
  [PlanningParameter] -> Specific Curve Trajectory Planning/3(PlanningParameter)
  Road data extraction/1(RoadLanePoly_Rotation) -> "Generate Road Lane from Polyfit TLC calculation "/2(PolyRoadLane)
  Road data extraction/2(RoadLaneEnd_Rotation) -> "Generate Road Lane from Polyfit TLC calculation "/3(RoadLaneEnd_Rotation)
  MATLAB Function1/1(TargetPath_VariableSize) -> TargetPath_Local/1
  MATLAB Function1/2(TargetSpeed_VariableSize) -> TargetSpeed_kmh/1
  Road data extraction/3(RoadLane_Plan) -> "Generate Road Lane from Polyfit TLC calculation "/1(RoadLane_Plan), Specific Curve Trajectory Planning/2(RoadLane_Plan), Out of Specific Curve Planning/1(RoadLane_Plan)

== system Prescan_Carsim_0118_repair_cs/BMW_X5_SUV_1/trajectory tracking Information ==
  note: Subsystem
  note: Preview Information Calculation
  TargetPath_Local : Inport
  TargetSpeed_kmh : Inport  Port=2
  Analog Filter Design1 : dsparch4/Analog Filter Design  method=Butterworth  filttype=Lowpass  N=1  Wlo=15  Whi=80  Rp=2  Rs=40
  Analog Filter Design2 : dsparch4/Analog Filter Design  method=Butterworth  filttype=Lowpass  N=1  Wlo=35  Whi=80  Rp=2  Rs=40
  Analog Filter Design3 : dsparch4/Analog Filter Design  method=Butterworth  filttype=Lowpass  N=1  Wlo=35  Whi=80  Rp=2  Rs=40
  Bus Creator2 : BusCreator  Inputs=5
  Mux1 : Mux  Inputs=5
  Preview Information Calculation 2 : MATLAB Function  TreatAsAtomicUnit=on
      settings: AttributesFormatString=|
      | The calculated Offset is Not Accurate
      | HeadError_rad:positive means the vehicle heads
      | left to the target path
  Scope1 : Scope
  planned speed Scope : Scope
  DataUsedForTracking (PrescanToTarget) : Outport  SampleTime=1/20
      settings: AttributesFormatString=Sample Time 1/20Hz
  wires:
  TargetPath_Local/1 -> Preview Information Calculation 2/1(TargetPath_Local)  "PreviewDistance"
  TargetSpeed_kmh/1 -> Preview Information Calculation 2/2(TargetSpeed_Plan)  "Speed_Planned_kmh"
  Analog Filter Design2/1 -> Mux1/3, Bus Creator2/2  "HeadError_rad"
  Analog Filter Design1/1 -> Mux1/2, Bus Creator2/1  "Preview Error"
  Preview Information Calculation 2/1(Offset_Preview) -> Analog Filter Design1/1  "Before Filter"
  Preview Information Calculation 2/2(HeadError_rad) -> Analog Filter Design2/1
  Preview Information Calculation 2/5(PreviewDistance) -> Bus Creator2/4  "PreviewDistance"
  Preview Information Calculation 2/4(TrackingError) -> Mux1/5
  Bus Creator2/1 -> DataUsedForTracking (PrescanToTarget)/1
  Mux1/1 -> planned speed Scope/1
  Preview Information Calculation 2/6(TargetSpeed_Current) -> Bus Creator2/5, Scope1/1  "Speed_Kmh"
  [Curve_Flag] -> Mux1/1
  Preview Information Calculation 2/3(Curvature_Vehicle) -> Analog Filter Design3/1
  Analog Filter Design3/1 -> Bus Creator2/3, Mux1/4  "Curvature"

== system Prescan_Carsim_0118_repair_cs/SteeringWheel_pivot_BMW_X5_SUV_1/Actuator ==
  Joint : Inport
  Bus Selector : BusSelector  OutputSignals=POSITION,ORIENTATION
  visu_Rotate : Subsystem  mask(RPYActuator){UniqueID=UniqueID, Object3DID=Rotate_ObjectID3D, TimeStep=TimeStep}
      mask prompts: UniqueID "Auto-Assigned: Unique ID"; Object3DID "Auto-Assigned: Child 3D Object ID"; TimeStep "Auto-Assigned: Upload Period [s]"
      mask help: Applies angles update to selected child object
      mask Help:
      | Applies position update to selected child object
      | 
      | - UniqueID (double)   : Unique ID of the parent actor
      | - Object3DID (string) : Name of the child 3D object
      mask Display: port_label('input', 1, ['visu_Rotate_' Object3DID])
  visu_Translate : Subsystem  mask(PositionActuator){UniqueID=UniqueID, Object3DID=Translate_ObjectID3D, TimeStep=TimeStep}
      mask prompts: UniqueID "Auto-Assigned: Unique ID"; Object3DID "Auto-Assigned: Child 3D Object ID"; TimeStep "Auto-Assigned: Upload Period [s]"
      mask help: Applies position update to selected child object
      mask Help:
      | Applies position update to selected child object
      | 
      | - UniqueID (double)   : Unique ID of the parent actor
      | - Object3DID (string) : Name of the child 3D object
      mask Display: port_label('input', 1, ['visu_Translate_' Object3DID])
  wires:
  Bus Selector/2 -> visu_Rotate/1(In1)  "<ORIENTATION>"
  Bus Selector/1 -> visu_Translate/1(In1)  "<POSITION>"
  Joint/1 -> Bus Selector/1

== system Prescan_Carsim_0118_repair_cs/WheelL0_BMW_X5_SUV_1/Actuator ==
  Joint : Inport
  Bus Selector : BusSelector  OutputSignals=POSITION,ORIENTATION
  visu_Rotate : Subsystem  mask(RPYActuator){UniqueID=UniqueID, Object3DID=Rotate_ObjectID3D, TimeStep=TimeStep}
      mask prompts: UniqueID "Auto-Assigned: Unique ID"; Object3DID "Auto-Assigned: Child 3D Object ID"; TimeStep "Auto-Assigned: Upload Period [s]"
      mask help: Applies angles update to selected child object
      mask Help:
      | Applies position update to selected child object
      | 
      | - UniqueID (double)   : Unique ID of the parent actor
      | - Object3DID (string) : Name of the child 3D object
      mask Display: port_label('input', 1, ['visu_Rotate_' Object3DID])
  visu_Translate : Subsystem  mask(PositionActuator){UniqueID=UniqueID, Object3DID=Translate_ObjectID3D, TimeStep=TimeStep}
      mask prompts: UniqueID "Auto-Assigned: Unique ID"; Object3DID "Auto-Assigned: Child 3D Object ID"; TimeStep "Auto-Assigned: Upload Period [s]"
      mask help: Applies position update to selected child object
      mask Help:
      | Applies position update to selected child object
      | 
      | - UniqueID (double)   : Unique ID of the parent actor
      | - Object3DID (string) : Name of the child 3D object
      mask Display: port_label('input', 1, ['visu_Translate_' Object3DID])
  wires:
  Bus Selector/2 -> visu_Rotate/1(In1)  "<ORIENTATION>"
  Bus Selector/1 -> visu_Translate/1(In1)  "<POSITION>"
  Joint/1 -> Bus Selector/1

== system Prescan_Carsim_0118_repair_cs/WheelL1_BMW_X5_SUV_1/Actuator ==
  Joint : Inport
  Bus Selector : BusSelector  OutputSignals=POSITION,ORIENTATION
  visu_Rotate : Subsystem  mask(RPYActuator){UniqueID=UniqueID, Object3DID=Rotate_ObjectID3D, TimeStep=TimeStep}
      mask prompts: UniqueID "Auto-Assigned: Unique ID"; Object3DID "Auto-Assigned: Child 3D Object ID"; TimeStep "Auto-Assigned: Upload Period [s]"
      mask help: Applies angles update to selected child object
      mask Help:
      | Applies position update to selected child object
      | 
      | - UniqueID (double)   : Unique ID of the parent actor
      | - Object3DID (string) : Name of the child 3D object
      mask Display: port_label('input', 1, ['visu_Rotate_' Object3DID])
  visu_Translate : Subsystem  mask(PositionActuator){UniqueID=UniqueID, Object3DID=Translate_ObjectID3D, TimeStep=TimeStep}
      mask prompts: UniqueID "Auto-Assigned: Unique ID"; Object3DID "Auto-Assigned: Child 3D Object ID"; TimeStep "Auto-Assigned: Upload Period [s]"
      mask help: Applies position update to selected child object
      mask Help:
      | Applies position update to selected child object
      | 
      | - UniqueID (double)   : Unique ID of the parent actor
      | - Object3DID (string) : Name of the child 3D object
      mask Display: port_label('input', 1, ['visu_Translate_' Object3DID])
  wires:
  Bus Selector/2 -> visu_Rotate/1(In1)  "<ORIENTATION>"
  Bus Selector/1 -> visu_Translate/1(In1)  "<POSITION>"
  Joint/1 -> Bus Selector/1

== system Prescan_Carsim_0118_repair_cs/WheelR0_BMW_X5_SUV_1/Actuator ==
  Joint : Inport
  Bus Selector : BusSelector  OutputSignals=POSITION,ORIENTATION
  visu_Rotate : Subsystem  mask(RPYActuator){UniqueID=UniqueID, Object3DID=Rotate_ObjectID3D, TimeStep=TimeStep}
      mask prompts: UniqueID "Auto-Assigned: Unique ID"; Object3DID "Auto-Assigned: Child 3D Object ID"; TimeStep "Auto-Assigned: Upload Period [s]"
      mask help: Applies angles update to selected child object
      mask Help:
      | Applies position update to selected child object
      | 
      | - UniqueID (double)   : Unique ID of the parent actor
      | - Object3DID (string) : Name of the child 3D object
      mask Display: port_label('input', 1, ['visu_Rotate_' Object3DID])
  visu_Translate : Subsystem  mask(PositionActuator){UniqueID=UniqueID, Object3DID=Translate_ObjectID3D, TimeStep=TimeStep}
      mask prompts: UniqueID "Auto-Assigned: Unique ID"; Object3DID "Auto-Assigned: Child 3D Object ID"; TimeStep "Auto-Assigned: Upload Period [s]"
      mask help: Applies position update to selected child object
      mask Help:
      | Applies position update to selected child object
      | 
      | - UniqueID (double)   : Unique ID of the parent actor
      | - Object3DID (string) : Name of the child 3D object
      mask Display: port_label('input', 1, ['visu_Translate_' Object3DID])
  wires:
  Bus Selector/2 -> visu_Rotate/1(In1)  "<ORIENTATION>"
  Bus Selector/1 -> visu_Translate/1(In1)  "<POSITION>"
  Joint/1 -> Bus Selector/1

== system Prescan_Carsim_0118_repair_cs/WheelR1_BMW_X5_SUV_1/Actuator ==
  Joint : Inport
  Bus Selector : BusSelector  OutputSignals=POSITION,ORIENTATION
  visu_Rotate : Subsystem  mask(RPYActuator){UniqueID=UniqueID, Object3DID=Rotate_ObjectID3D, TimeStep=TimeStep}
      mask prompts: UniqueID "Auto-Assigned: Unique ID"; Object3DID "Auto-Assigned: Child 3D Object ID"; TimeStep "Auto-Assigned: Upload Period [s]"
      mask help: Applies angles update to selected child object
      mask Help:
      | Applies position update to selected child object
      | 
      | - UniqueID (double)   : Unique ID of the parent actor
      | - Object3DID (string) : Name of the child 3D object
      mask Display: port_label('input', 1, ['visu_Rotate_' Object3DID])
  visu_Translate : Subsystem  mask(PositionActuator){UniqueID=UniqueID, Object3DID=Translate_ObjectID3D, TimeStep=TimeStep}
      mask prompts: UniqueID "Auto-Assigned: Unique ID"; Object3DID "Auto-Assigned: Child 3D Object ID"; TimeStep "Auto-Assigned: Upload Period [s]"
      mask help: Applies position update to selected child object
      mask Help:
      | Applies position update to selected child object
      | 
      | - UniqueID (double)   : Unique ID of the parent actor
      | - Object3DID (string) : Name of the child 3D object
      mask Display: port_label('input', 1, ['visu_Translate_' Object3DID])
  wires:
  Bus Selector/2 -> visu_Rotate/1(In1)  "<ORIENTATION>"
  Bus Selector/1 -> visu_Translate/1(In1)  "<POSITION>"
  Joint/1 -> Bus Selector/1

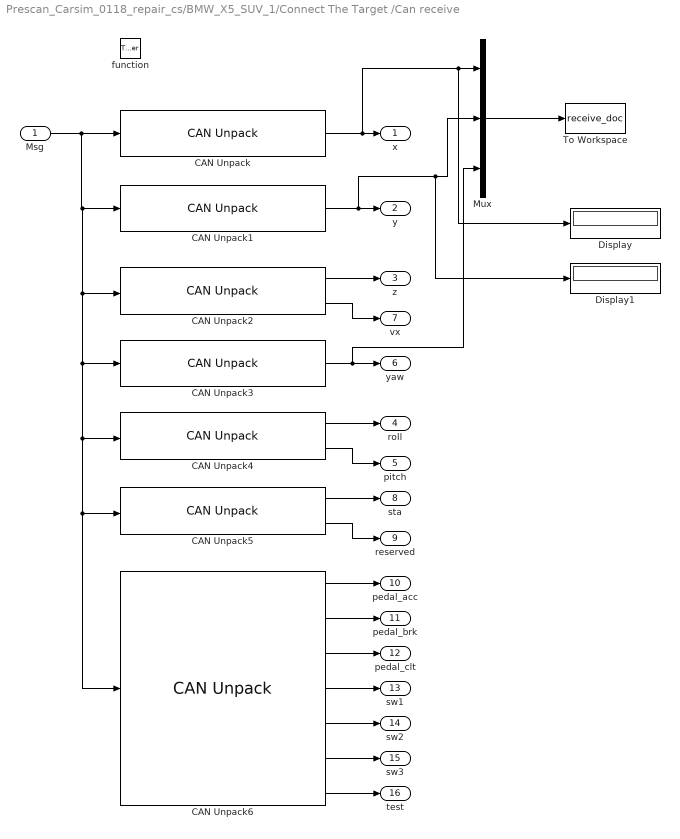
== system Prescan_Carsim_0118_repair_cs/BMW_X5_SUV_1/Connect The Target /Can receive ==
  Msg : Inport
  function : TriggerPort  TriggerType=function-call  VariantControl=Variant
  CAN Unpack : canmsglib/CAN Unpack  MsgList=(none)  MsgName=CAN Msg  MsgIDType=Standard (11-bit identifier)  MsgIdentifier=100  MsgLength=8  SignalInfo={'x','0','64','LE','double','Standard','0','1','0','-Inf','Inf'}  IDPort=off  TimestampPort=off  ErrorPort=off  RemotePort=off  LengthPort=off  StatusPort=off  ApplyMinMax=off
      settings: SourceProductName=Simulink Real-Time  SourceProductBaseCode=XP
  CAN Unpack1 : canmsglib/CAN Unpack  MsgList=(none)  MsgName=CAN Msg  MsgIDType=Standard (11-bit identifier)  MsgIdentifier=101  MsgLength=8  SignalInfo={'y','0','64','LE','double','Standard','0','1','0','-Inf','Inf'}  IDPort=off  TimestampPort=off  ErrorPort=off  RemotePort=off  LengthPort=off  StatusPort=off  ApplyMinMax=off
      settings: SourceProductName=Simulink Real-Time  SourceProductBaseCode=XP
  CAN Unpack2 : canmsglib/CAN Unpack  MsgList=(none)  MsgName=CAN Msg  MsgIDType=Standard (11-bit identifier)  MsgIdentifier=102  MsgLength=8  SignalInfo={'z','0','32','LE','single','Standard','0','1','0','-Inf','Inf';'vx','32','32','LE','single','Standard','0','1','0','-Inf','Inf'}  IDPort=off  TimestampPort=off  ErrorPort=off  RemotePort=off  LengthPort=off  StatusPort=off  ApplyMinMax=off
      settings: SourceProductName=Simulink Real-Time  SourceProductBaseCode=XP
  CAN Unpack3 : canmsglib/CAN Unpack  MsgList=(none)  MsgName=CAN Msg  MsgIDType=Standard (11-bit identifier)  MsgIdentifier=103  MsgLength=8  SignalInfo={'yaw','0','64','LE','double','Standard','0','1','0','-Inf','Inf'}  IDPort=off  TimestampPort=off  ErrorPort=off  RemotePort=off  LengthPort=off  StatusPort=off  ApplyMinMax=off
      settings: SourceProductName=Simulink Real-Time  SourceProductBaseCode=XP
  CAN Unpack4 : canmsglib/CAN Unpack  MsgList=(none)  MsgName=CAN Msg  MsgIDType=Standard (11-bit identifier)  MsgIdentifier=104  MsgLength=8  SignalInfo={'roll','0','32','LE','single','Standard','0','1','0','-Inf','Inf';'pitch','32','32','LE','single','Standard','0','1','0','-Inf','Inf'}  IDPort=off  TimestampPort=off  ErrorPort=off  RemotePort=off  LengthPort=off  StatusPort=off  ApplyMinMax=off
      settings: SourceProductName=Simulink Real-Time  SourceProductBaseCode=XP
  CAN Unpack5 : canmsglib/CAN Unpack  MsgList=(none)  MsgName=CAN Msg  MsgIDType=Standard (11-bit identifier)  MsgIdentifier=105  MsgLength=8  SignalInfo={'sta','0','32','LE','single','Standard','0','1','0','-Inf','Inf';'reserved','32','32','LE','single','Standard','0','1','0','-Inf','Inf'}  IDPort=off  TimestampPort=off  ErrorPort=off  RemotePort=off  LengthPort=off  StatusPort=off  ApplyMinMax=off
      settings: SourceProductName=Simulink Real-Time  SourceProductBaseCode=XP
  CAN Unpack6 : canmsglib/CAN Unpack  MsgList=(none)  MsgName=CAN Msg  MsgIDType=Standard (11-bit identifier)  MsgIdentifier=106  MsgLength=8  SignalInfo={'pedal_acc','0','8','LE','unsigned','Standard','0','1','0','-Inf','Inf';'pedal_brk','8','8','LE','unsigned','Standard','0','1','0','-Inf','Inf';'pedal_clt','16','8','LE','unsigned','Standard','0','1','0','-Inf','Inf';'sw1','24','8','LE','unsigned','Standard','0','1','0','-Inf','Inf';'sw2','32','8','LE','unsigned','Standard','0','1','0','-Inf','Inf';'sw3','40','8','LE','unsigned','Standard','0','1','0','-Inf','Inf';'test','48','16','LE','unsigned','Standard','0','1','0','-Inf','Inf'}  IDPort=off  TimestampPort=off  ErrorPort=off  RemotePort=off  LengthPort=off  StatusPort=off  ApplyMinMax=off
      settings: SourceProductName=Simulink Real-Time  SourceProductBaseCode=XP
  Display : Display
  Display1 : Display
  Mux : Mux  Inputs=3
  To Workspace : ToWorkspace  VariableName=receive_doc  SaveFormat=Timeseries  SampleTime=-1
  x : Outport  VectorParamsAs1DForOutWhenUnconnected=off
  y : Outport  Port=2  VectorParamsAs1DForOutWhenUnconnected=off
  z : Outport  Port=3  VectorParamsAs1DForOutWhenUnconnected=off
  roll : Outport  Port=4  VectorParamsAs1DForOutWhenUnconnected=off
  pitch : Outport  Port=5  VectorParamsAs1DForOutWhenUnconnected=off
  yaw : Outport  Port=6  VectorParamsAs1DForOutWhenUnconnected=off
  vx : Outport  Port=7  VectorParamsAs1DForOutWhenUnconnected=off
  sta : Outport  Port=8  VectorParamsAs1DForOutWhenUnconnected=off
  reserved : Outport  Port=9  VectorParamsAs1DForOutWhenUnconnected=off
  pedal_acc : Outport  Port=10  VectorParamsAs1DForOutWhenUnconnected=off
  pedal_brk : Outport  Port=11  VectorParamsAs1DForOutWhenUnconnected=off
  pedal_clt : Outport  Port=12  VectorParamsAs1DForOutWhenUnconnected=off
  sw1 : Outport  Port=13  VectorParamsAs1DForOutWhenUnconnected=off
  sw2 : Outport  Port=14  VectorParamsAs1DForOutWhenUnconnected=off
  sw3 : Outport  Port=15  VectorParamsAs1DForOutWhenUnconnected=off
  test : Outport  Port=16  VectorParamsAs1DForOutWhenUnconnected=off
  wires:
  Mux/1 -> To Workspace/1
  CAN Unpack6/7 -> test/1
  CAN Unpack6/6 -> sw3/1
  CAN Unpack6/5 -> sw2/1
  CAN Unpack6/4 -> sw1/1
  CAN Unpack6/3 -> pedal_clt/1
  CAN Unpack6/2 -> pedal_brk/1
  CAN Unpack6/1 -> pedal_acc/1
  CAN Unpack5/2 -> reserved/1
  CAN Unpack5/1 -> sta/1
  CAN Unpack4/2 -> pitch/1
  CAN Unpack4/1 -> roll/1
  CAN Unpack3/1 -> yaw/1, Mux/3
  CAN Unpack2/2 -> vx/1
  CAN Unpack2/1 -> z/1
  CAN Unpack1/1 -> y/1, Display1/1, Mux/2
  CAN Unpack/1 -> x/1, Display/1, Mux/1
  Msg/1 -> CAN Unpack/1, CAN Unpack1/1, CAN Unpack2/1, CAN Unpack3/1, CAN Unpack4/1, CAN Unpack5/1, CAN Unpack6/1

== system Prescan_Carsim_0118_repair_cs/BMW_X5_SUV_1/Connect The Target /simple_filter10 ==
  In1 : Inport
  Add : Sum
  Gain10 : Gain  Gain=0.5
  Memory : Memory
  Out1 : Outport  VectorParamsAs1DForOutWhenUnconnected=off
  wires:
  Gain10/1 -> Out1/1
  Memory/1 -> Add/2
  In1/1 -> Add/1, Memory/1
  Add/1 -> Gain10/1

== system Prescan_Carsim_0118_repair_cs/BMW_X5_SUV_1/Connect The Target /simple_filter11 ==
  In1 : Inport
  Add : Sum
  Gain10 : Gain  Gain=0.5
  Memory : Memory
  Out1 : Outport  VectorParamsAs1DForOutWhenUnconnected=off
  wires:
  Gain10/1 -> Out1/1
  Memory/1 -> Add/2
  In1/1 -> Add/1, Memory/1
  Add/1 -> Gain10/1

== system Prescan_Carsim_0118_repair_cs/BMW_X5_SUV_1/Connect The Target /simple_filter6 ==
  In1 : Inport
  Add : Sum
  Gain10 : Gain  Gain=0.5
  Memory : Memory
  Out1 : Outport  VectorParamsAs1DForOutWhenUnconnected=off
  wires:
  Add/1 -> Gain10/1
  In1/1 -> Memory/1, Add/1
  Memory/1 -> Add/2
  Gain10/1 -> Out1/1

== system Prescan_Carsim_0118_repair_cs/BMW_X5_SUV_1/Connect The Target /simple_filter7 ==
  In1 : Inport
  Add : Sum
  Gain10 : Gain  Gain=0.5
  Memory : Memory
  Out1 : Outport  VectorParamsAs1DForOutWhenUnconnected=off
  wires:
  Gain10/1 -> Out1/1
  Memory/1 -> Add/2
  In1/1 -> Add/1, Memory/1
  Add/1 -> Gain10/1

== system Prescan_Carsim_0118_repair_cs/BMW_X5_SUV_1/Connect The Target /simple_filter8 ==
  In1 : Inport
  Add : Sum
  Gain10 : Gain  Gain=0.5
  Memory : Memory
  Out1 : Outport  VectorParamsAs1DForOutWhenUnconnected=off
  wires:
  Add/1 -> Gain10/1
  In1/1 -> Memory/1, Add/1
  Memory/1 -> Add/2
  Gain10/1 -> Out1/1

== system Prescan_Carsim_0118_repair_cs/BMW_X5_SUV_1/Connect The Target /simple_filter9 ==
  In1 : Inport
  Add : Sum
  Gain10 : Gain  Gain=0.5
  Memory : Memory
  Out1 : Outport  VectorParamsAs1DForOutWhenUnconnected=off
  wires:
  Gain10/1 -> Out1/1
  Memory/1 -> Add/2
  In1/1 -> Add/1, Memory/1
  Add/1 -> Gain10/1

== system Prescan_Carsim_0118_repair_cs/BMW_X5_SUV_1/Connect The Target /simplefilter ==
  In1 : Inport
  Add : Sum
  Gain : Gain  Gain=0.5
  Memory : Memory
  Out1 : Outport  VectorParamsAs1DForOutWhenUnconnected=off
  wires:
  Gain/1 -> Out1/1
  Memory/1 -> Add/2
  Add/1 -> Gain/1
  In1/1 -> Memory/1, Add/1
